simulink model "coord_rotations_test"  (R2016b)
settings: Solver=VariableStepAuto  StartTime=0.0  StopTime=10.0  RelTol=1e-3
libraries: coord_rotations_lib x2
settings Model: Creator=taylorreynolds  LastModifiedBy=taylorreynolds

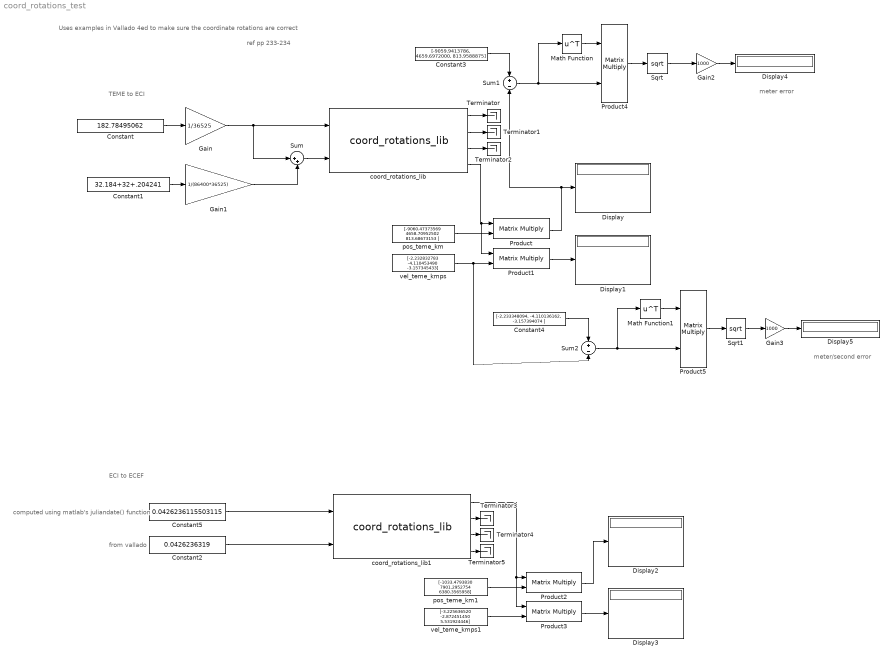
== system coord_rotations_test ==
  note: ref pp 233-234
  note: meter/second error
  note: meter error
  note: ECI to ECEF
  note: TEME to ECI
  note: Uses examples in Vallado 4ed to make sure the coordinate rotations are correct
  note: from vallado
  note: computed using matlab's juliandate() function
  Constant : Constant  Value=182.78495062
  Constant1 : Constant  Value=32.184+32+.204241
  Constant2 : Constant  Value=0.0426236319
  Constant3 : Constant  Value=[-9059.9413786, 4659.6972000, 813.9588875]
  Constant4 : Constant  Value=[-2.233348094, -4.110136162, -3.157394074 ]
  Constant5 : Constant  Value=0.0426236115503115
  Display{,1..5} (6 alike) : Display
  Gain : Gain  Gain=1/36525
  Gain1 : Gain  Gain=1/(86400*36525)
  Gain2 : Gain  Gain=1000
  Gain3 : Gain  Gain=1000
  Math Function : Math  Operator=transpose  SaturateOnIntegerOverflow=on
  Math Function1 : Math  Operator=transpose  SaturateOnIntegerOverflow=on
  Product{,1..5} (6 alike) : Product  Multiplication=Matrix(*)
  Sqrt : Sqrt  SaturateOnIntegerOverflow=on
  Sqrt1 : Sqrt  SaturateOnIntegerOverflow=on
  Sum : Sum  Inputs=|++
  Sum1 : Sum  Inputs=+-
  Sum2 : Sum  Inputs=+-
  Terminator{,1..5} (6 alike) : Terminator
  coord_rotations_lib : coord_rotations_lib/coord_rotations_lib
  coord_rotations_lib1 : coord_rotations_lib/coord_rotations_lib
  pos_teme_km : Constant  Value=[-9060.47373569 4658.70952502 813.68673153 ]
  pos_teme_km1 : Constant  Value=[-1033.4793830 7901.2952754 6380.3565958]
  vel_teme_kmps : Constant  Value=[-2.232832783 -4.110453490 -3.157345433]
  vel_teme_kmps1 : Constant  Value=[-3.225636520 -2.872451450 5.531924446]
  wires:
  Constant/1 -> Gain/1
  Gain/1 -> Sum/1, coord_rotations_lib/1
  Constant1/1 -> Gain1/1
  Gain1/1 -> Sum/2
  Sum/1 -> coord_rotations_lib/2
  coord_rotations_lib/1 -> Terminator/1
  coord_rotations_lib/3 -> Terminator2/1
  coord_rotations_lib/2 -> Terminator1/1
  coord_rotations_lib/4 -> Product1/1, Product/1
  pos_teme_km/1 -> Product/2
  vel_teme_kmps/1 -> Sum2/2, Product1/2
  Product/1 -> Display/1, Sum1/2
  Product1/1 -> Display1/1
  Constant2/1 -> coord_rotations_lib1/2
  Constant5/1 -> coord_rotations_lib1/1
  pos_teme_km1/1 -> Product2/2
  vel_teme_kmps1/1 -> Product3/2
  Product2/1 -> Display2/1
  Product3/1 -> Display3/1
  coord_rotations_lib1/2 -> Terminator3/1
  coord_rotations_lib1/3 -> Terminator4/1
  coord_rotations_lib1/4 -> Terminator5/1
  coord_rotations_lib1/1 -> Product3/1, Product2/1
  Constant3/1 -> Sum1/1
  Sum1/1 -> Math Function/1, Product4/2
  Math Function/1 -> Product4/1
  Product4/1 -> Sqrt/1
  Sqrt/1 -> Gain2/1
  Constant4/1 -> Sum2/1
  Sum2/1 -> Math Function1/1, Product5/2
  Math Function1/1 -> Product5/1
  Product5/1 -> Sqrt1/1
  Sqrt1/1 -> Gain3/1
  Gain2/1 -> Display4/1
  Gain3/1 -> Display5/1
